simulink model "example_of_compare_to_constant"  (R2021a)
settings: Solver=VariableStepAuto  StartTime=0.0  StopTime=10.0  MaxStep=1e-3  RelTol=1e-3
libraries: simulink x3
settings Model: Creator=YasserNet  LastModifiedBy=YasserNet

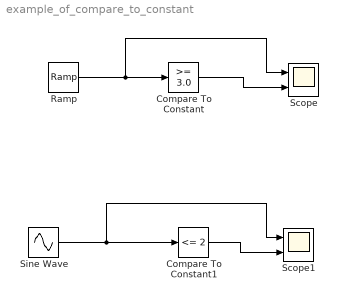
== system example_of_compare_to_constant ==
  Compare To Constant : simulink/Logic and Bit Operations/Compare To Constant  relop=>=  const=3.0  OutDataTypeStr=boolean
  Compare To Constant1 : simulink/Logic and Bit Operations/Compare To Constant  relop=<=  const=2  OutDataTypeStr=boolean
  Ramp : simulink/Sources/Ramp  slope=1  start=2  InitialOutput=-0.5
  Scope : Scope  NumInputPorts=2
  Scope1 : Scope  NumInputPorts=2
  Sine Wave : Sin  Amplitude=10  Frequency=2*pi*3  SampleTime=0
  wires:
  Compare To Constant1/1 -> Scope1/2
  Ramp/1 -> Compare To Constant/1, Scope/1
  Sine Wave/1 -> Compare To Constant1/1, Scope1/1
  Compare To Constant/1 -> Scope/2
